simulink model "modelBallPumpDualAction"  (R2021a)
settings: Solver=VariableStepAuto  StartTime=0.0  StopTime=60  RelTol=1e-5  AbsTol=1e-5
PreLoadFcn:
  | paramBallPump;
values from neighbouring files (symbols this model uses):
  area1_pump2 = pi*(diameter1_pump2/2)^2    (= 380.132711084)    [paramBallPump.m]
  area2_pump2 = pi*(diameter1_pump2/2)^2 - pi*(diameter2_pump2/2)^2    (= 301.592894745)    [paramBallPump.m]
  area_valve = pi*(diameter_valve/2)^2    (= 3.14159265359)    [paramBallPump.m]
  pdiff_valve = 1000    [paramBallPump.m]
  stroke_pump2 = 105    [paramBallPump.m]
libraries: fl_lib x17, SimscapeFluids_lib x4, nesl_utility x2
settings Model: Creator=ytang  LastModifiedBy=ytang
settings SolverCC: AutoScaleAbsTol=off  AlgebraicLoopSolver=TrustRegion
settings DebuggingCC: SymbolicDimsDataTypeCodeGenerationDiagnostic=none  SFMachineParentedDataDiag=warning
settings SFSimCC: CustomCodeUndefinedFunction=UseInterfaceOnly
settings SimscapeCC: SimscapeLogType=all  SimscapeLogOpenViewer=on  SimscapeLogLimitData=off  SimscapeLogDataHistory=10000

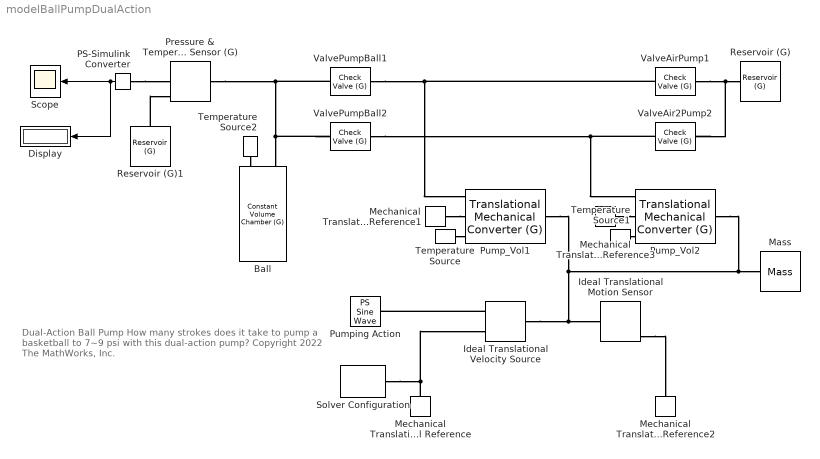
== system modelBallPumpDualAction ==
  note: Dual-Action Ball Pump
      |
      | How many strokes does it take to pump a basketball
      | to 7~9 psi with this dual-action pump?
      |
      | Copyright 2022 The MathWorks, Inc.
  Ball : fl_lib/Gas/Elements/Constant Volume Chamber (G)  volume=volume_ball mm^3  num_ports=foundation.enum.num_ports.one  area_A=1 mm^2  area_B=0.01 m^2  area_C=0.01 m^2  area_D=0.01 m^2  p_I_specify=off  p_I_priority=High  p_I=0.101325 MPa  p_I_nominal_specify=off  p_I_nominal_unit=MPa  p_I_nominal_value=1  T_I_specify=off  T_I_priority=High  T_I=293.15 K  T_I_nominal_specify=off  T_I_nominal_unit=K  T_I_nominal_value=1  rho_chamber_specify=off  rho_chamber_priority=None  rho_chamber=1.2 kg/m^3  rho_chamber_nominal_specify=off  rho_chamber_nominal_unit=kg/m^3  rho_chamber_nominal_value=1
      settings: SourceProductBaseCode=SS  InternalSimscapePortConfiguration="{\"Bottom\":[],\"Left\":[{\"id\":\"A\",\"label\":\"A\",\"type\":\"foundation.gas.gas\"},{\"id\":\"H\",\"label\":\"H\",\"type\":\"foundation.thermal.thermal\"}],\"Right\":[],\"Top\":[]}"
  Display : Display
  Ideal Translational Motion Sensor : fl_lib/Mechanical/Mechanical Sensors/Ideal Translational Motion Sensor  offset=0 m
  Ideal Translational Velocity Source : fl_lib/Mechanical/Mechanical Sources/Ideal Translational Velocity Source
  Mass : fl_lib/Mechanical/Translational Elements/Mass  mass=mass_pump2 g  num_ports=foundation.enum.numPorts2.one  v_specify=off  v_priority=High  v=0 m/s  v_nominal_specify=off  v_nominal_unit=m/s  v_nominal_value=1  f_specify=off  f_priority=None  f=0 N  f_nominal_specify=off  f_nominal_unit=N  f_nominal_value=1
  Mechanical Translational Reference{,1..3} (4 alike) : fl_lib/Mechanical/Translational Elements/Mechanical Translational Reference
  PS-Simulink Converter : nesl_utility/PS-Simulink Converter  PhysicalDomain=network_engine_domain  SubClassName=ps_output  LeftPortType=input  RightPortType=output  PseudoPeriodic=off  Frequencies=[]  Unit=psi  AffineConversion=off
      settings: SourceProductBaseCode=PW,SS
  Pressure & Temperature Sensor (G) : fl_lib/Gas/Sensors/Pressure & Temperature Sensor (G)
      settings: SourceProductBaseCode=SS  InternalSimscapePortConfiguration="{\"Bottom\":[],\"Left\":[{\"id\":\"A\",\"label\":\"A\",\"type\":\"foundation.gas.gas\"}],\"Right\":[{\"id\":\"B\",\"label\":\"B\",\"type\":\"foundation.gas.gas\"},{\"id\":\"P\",\"label\":\"P\",\"type\":\"output\"},{\"id\":\"T\",\"label\":\"T\",\"type\":\"output\"}],\"Top\":[]}"
  Pump_Vol1 : fl_lib/Gas/Elements/Translational Mechanical Converter (G)  mech_orientation=foundation.enum.MechOrientationTranslational.Positive  displacement_spec=foundation.enum.DisplacementSpec.Calculate  length_init=0 m  interface_area=area1_pump2 mm^2  dead_volume=endvolume1_pump2 mm^3  area_A=area1_pump2 * 1.2 mm^2  environment_spec=foundation.enum.pressure_spec.atmospheric  environment_pressure=0.101325 MPa  p_I_specify=off  p_I_priority=High  p_I=0.101325 MPa  p_I_nominal_specify=off  p_I_nominal_unit=MPa  p_I_nominal_value=1  T_I_specify=off  T_I_priority=High  T_I=293.15 K  T_I_nominal_specify=off  T_I_nominal_unit=K  T_I_nominal_value=1  rho_converter_specify=off  rho_converter_priority=None  rho_converter=1.2 kg/m^3  rho_converter_nominal_specify=off  rho_converter_nominal_unit=kg/m^3  rho_converter_nominal_value=1
      settings: SourceProductBaseCode=SS  InternalSimscapePortConfiguration="{\"Bottom\":[],\"Left\":[{\"id\":\"A\",\"label\":\"A\",\"type\":\"foundation.gas.gas\"},{\"id\":\"C\",\"label\":\"C\",\"type\":\"foundation.mechanical.translational.translational\"},{\"id\":\"H\",\"label\":\"H\",\"type\":\"foundation.thermal.thermal\"}],\"Right\":[{\"id\":\"R\",\"label\":\"R\",\"type\":\"foundation.mechanical.translational.translational\"}],\"Top\":[]}"
  Pump_Vol2 : fl_lib/Gas/Elements/Translational Mechanical Converter (G)  mech_orientation=foundation.enum.MechOrientationTranslational.Negative  displacement_spec=foundation.enum.DisplacementSpec.Calculate  length_init=-stroke_pump2 mm  interface_area=area2_pump2 mm^2  dead_volume=endvolume2_pump2 mm^3  area_A=area2_pump2 * 1.2 mm^2  environment_spec=foundation.enum.pressure_spec.atmospheric  environment_pressure=0.101325 MPa  p_I_specify=off  p_I_priority=High  p_I=0.101325 MPa  p_I_nominal_specify=off  p_I_nominal_unit=MPa  p_I_nominal_value=1  T_I_specify=off  T_I_priority=High  T_I=293.15 K  T_I_nominal_specify=off  T_I_nominal_unit=K  T_I_nominal_value=1  rho_converter_specify=off  rho_converter_priority=None  rho_converter=1.2 kg/m^3  rho_converter_nominal_specify=off  rho_converter_nominal_unit=kg/m^3  rho_converter_nominal_value=1
      settings: SourceProductBaseCode=SS  InternalSimscapePortConfiguration="{\"Bottom\":[],\"Left\":[{\"id\":\"A\",\"label\":\"A\",\"type\":\"foundation.gas.gas\"},{\"id\":\"C\",\"label\":\"C\",\"type\":\"foundation.mechanical.translational.translational\"},{\"id\":\"H\",\"label\":\"H\",\"type\":\"foundation.thermal.thermal\"}],\"Right\":[{\"id\":\"R\",\"label\":\"R\",\"type\":\"foundation.mechanical.translational.translational\"}],\"Top\":[]}"
  Pumping Action : fl_lib/Physical Signals/Sources/PS Sine Wave  amplitude=amplitude_pump2 mm/s  bias=0 m/s  frequency_spec=foundation.enum.frequencySpec.frequencySI  frequency_SI=frequency_pump2 Hz  frequency_angular=1 rad/s  phase=0 rad
      settings: SourceProductBaseCode=SS  InternalSimscapePortConfiguration="{\"Bottom\":[],\"Left\":[],\"Right\":[{\"id\":\"O\",\"label\":\"\",\"type\":\"output\"}],\"Top\":[]}"
  Reservoir (G) : fl_lib/Gas/Elements/Reservoir (G)  pressure_spec=foundation.enum.pressure_spec.atmospheric  reservoir_pressure=0.101325 MPa  reservoir_temperature=293.15 K  area_A=area_valve * 2 mm^2
      settings: SourceProductBaseCode=SS
  Reservoir (G)1 : fl_lib/Gas/Elements/Reservoir (G)  pressure_spec=foundation.enum.pressure_spec.atmospheric  reservoir_pressure=0.101325 MPa  reservoir_temperature=293.15 K  area_A=area_valve * 2 mm^2
      settings: SourceProductBaseCode=SS
  Scope : Scope
  Solver Configuration : nesl_utility/Solver Configuration  PhysicalDomain=network_engine_domain  SubClassName=solver  LeftPortType=input  RightPortType=generic  Tones=[]  Harmonics=[]  SimulateNoise=off  Profile=off  UseLocalSampling=off  EnableSwitchedLinearOptims=on  FrequencyDomain=off  UseCCode=off  RelTol=0.001  AbsTol=1e-06  MinStep=1e-09  ToWorkspace=off  RevertToSquareIcSolve=off  NumHomotopyIterations=100  PhasorMode=off  PhasorModeNumHarmonics=1  DoDC=off  ResidualTolerance=1e-09  UseLocalSolver=off  LocalSolverChoice=NE_BACKWARD_EULER_ADVANCER  LocalSolverSampleTime=0.001  DoFixedCost=off  MaxNonlinIter=3  MaxModeIter=2  ComputeImpulses=off  ImpulseIterations=2  LinearAlgebra=auto  EquationFormulation=NE_TIME_EF  DelaysMemoryBudget=1024  AutomaticFiltering=on  FilteringTimeConstant=0.001  PartitionStorageMethod=AS_NEEDED  PartitionMemoryBudget=1024  PartitionMethod=ROBUST
      settings: SourceProductBaseCode=PW,SS
  Temperature Source : fl_lib/Thermal/Thermal Sources/Temperature Source  temperature=293.15 K
  Temperature Source1 : fl_lib/Thermal/Thermal Sources/Temperature Source  temperature=293.15 K
  Temperature Source2 : fl_lib/Thermal/Thermal Sources/Temperature Source  temperature=293.15 K
  ValveAir2Pump2 : SimscapeFluids_lib/Gas/Valves & Orifices/Directional Control Valves/Check Valve (G)  pressure_spec=fluids.gas.enum.pressure_control_spec.dp  p_crack_differential=pdiff_valve Pa  p_crack_gauge=0.1 MPa  press_max_differential=pdiff_valve * 1.2 Pa  press_max_gauge=0.2 MPa  iso_cond_spec=fluids.gas.enum.iso_cond_spec.area  C_max=1.6 l/s/bar  C_min=1e-5 l/s/bar  B_crit=0.3  m=0.5  Cv_max=0.4  Cv_min=1e-6  Kv_max=0.3  Kv_min=1e-6  area_max=area_valve mm^2  area_leak=1e-12 m^2  area=area_valve * 2 mm^2  smoothing_factor=0  B_lam=0.999  T0=293.15 K  rho0=1.185 kg/m^3
      settings: SourceProductBaseCode=SH  InternalSimscapePortConfiguration="{\"Bottom\":[],\"Left\":[{\"id\":\"A\",\"label\":\"A\",\"type\":\"foundation.gas.gas\"}],\"Right\":[{\"id\":\"B\",\"label\":\"B\",\"type\":\"foundation.gas.gas\"}],\"Top\":[]}"
  ValveAirPump1 : SimscapeFluids_lib/Gas/Valves & Orifices/Directional Control Valves/Check Valve (G)  pressure_spec=fluids.gas.enum.pressure_control_spec.dp  p_crack_differential=pdiff_valve Pa  p_crack_gauge=0.1 MPa  press_max_differential=pdiff_valve * 1.2 Pa  press_max_gauge=0.2 MPa  iso_cond_spec=fluids.gas.enum.iso_cond_spec.area  C_max=1.6 l/s/bar  C_min=1e-5 l/s/bar  B_crit=0.3  m=0.5  Cv_max=0.4  Cv_min=1e-6  Kv_max=0.3  Kv_min=1e-6  area_max=area_valve mm^2  area_leak=1e-12 m^2  area=area_valve * 2 mm^2  smoothing_factor=0  B_lam=0.999  T0=293.15 K  rho0=1.185 kg/m^3
      settings: SourceProductBaseCode=SH  InternalSimscapePortConfiguration="{\"Bottom\":[],\"Left\":[{\"id\":\"A\",\"label\":\"A\",\"type\":\"foundation.gas.gas\"}],\"Right\":[{\"id\":\"B\",\"label\":\"B\",\"type\":\"foundation.gas.gas\"}],\"Top\":[]}"
  ValvePumpBall1 : SimscapeFluids_lib/Gas/Valves & Orifices/Directional Control Valves/Check Valve (G)  pressure_spec=fluids.gas.enum.pressure_control_spec.dp  p_crack_differential=pdiff_valve Pa  p_crack_gauge=0.1 MPa  press_max_differential=pdiff_valve * 1.2 Pa  press_max_gauge=0.2 MPa  iso_cond_spec=fluids.gas.enum.iso_cond_spec.area  C_max=1.6 l/s/bar  C_min=1e-5 l/s/bar  B_crit=0.3  m=0.5  Cv_max=0.4  Cv_min=1e-6  Kv_max=0.3  Kv_min=1e-6  area_max=area_valve mm^2  area_leak=1e-12 m^2  area=area_valve * 2 mm^2  smoothing_factor=0  B_lam=0.999  T0=293.15 K  rho0=1.185 kg/m^3
      settings: SourceProductBaseCode=SH  InternalSimscapePortConfiguration="{\"Bottom\":[],\"Left\":[{\"id\":\"A\",\"label\":\"A\",\"type\":\"foundation.gas.gas\"}],\"Right\":[{\"id\":\"B\",\"label\":\"B\",\"type\":\"foundation.gas.gas\"}],\"Top\":[]}"
  ValvePumpBall2 : SimscapeFluids_lib/Gas/Valves & Orifices/Directional Control Valves/Check Valve (G)  pressure_spec=fluids.gas.enum.pressure_control_spec.dp  p_crack_differential=pdiff_valve Pa  p_crack_gauge=0.1 MPa  press_max_differential=pdiff_valve * 1.2 Pa  press_max_gauge=0.2 MPa  iso_cond_spec=fluids.gas.enum.iso_cond_spec.area  C_max=1.6 l/s/bar  C_min=1e-5 l/s/bar  B_crit=0.3  m=0.5  Cv_max=0.4  Cv_min=1e-6  Kv_max=0.3  Kv_min=1e-6  area_max=area_valve mm^2  area_leak=1e-12 m^2  area=area_valve * 2 mm^2  smoothing_factor=0  B_lam=0.999  T0=293.15 K  rho0=1.185 kg/m^3
      settings: SourceProductBaseCode=SH  InternalSimscapePortConfiguration="{\"Bottom\":[],\"Left\":[{\"id\":\"A\",\"label\":\"A\",\"type\":\"foundation.gas.gas\"}],\"Right\":[{\"id\":\"B\",\"label\":\"B\",\"type\":\"foundation.gas.gas\"}],\"Top\":[]}"
  wires:
  PS-Simulink Converter/1 -> Display/1, Scope/1
  connections:
  Ideal Translational Velocity Source/RConn1 -- Pumping Action/RConn1
  Mechanical Translational Reference/LConn1 -- Ideal Translational Velocity Source/RConn2 -- Solver Configuration/RConn1
  Ideal Translational Velocity Source/LConn1 -- Pump_Vol1/RConn1 -- Pump_Vol2/RConn1 -- Mass/LConn1 -- Ideal Translational Motion Sensor/LConn1
  Mechanical Translational Reference1/LConn1 -- Pump_Vol1/LConn2
  ValvePumpBall1/RConn1 -- Pressure & Temperature Sensor (G)/LConn1 -- Ball/LConn1 -- ValvePumpBall2/RConn1
  ValveAirPump1/RConn1 -- ValvePumpBall1/LConn1 -- Pump_Vol1/LConn1
  ValveAirPump1/LConn1 -- ValveAir2Pump2/LConn1 -- Reservoir (G)/LConn1
  PS-Simulink Converter/LConn1 -- Pressure & Temperature Sensor (G)/RConn2
  Reservoir (G)1/LConn1 -- Pressure & Temperature Sensor (G)/RConn1
  Ideal Translational Motion Sensor/RConn1 -- Mechanical Translational Reference2/LConn1
  Mechanical Translational Reference3/LConn1 -- Pump_Vol2/LConn2
  ValvePumpBall2/LConn1 -- ValveAir2Pump2/RConn1 -- Pump_Vol2/LConn1
  Temperature Source/LConn1 -- Pump_Vol1/LConn3
  Temperature Source1/LConn1 -- Pump_Vol2/LConn3
  Temperature Source2/LConn1 -- Ball/LConn2
